simulink model "PHRControl"  (R2022a)
settings: Solver=FixedStepAuto  StartTime=0.0  StopTime=inf  FixedStep=.005  RelTol=1e-3
model workspace (MAT data in the model file):
  CPR = 10000
  amplitude = 0
  contactTime = 0
  desired_speed = 0
  equilibrium_length = 0
  h = 35
  hip_bend_factor = 0
  hip_fuzz = 0
  initHip = 0.523598775598
  initKnee = -1.0471975512
  k_landing_angle = 0
  k_slip = 0
  knee_bend_factor = 0
  knee_fuzz = 0
  lower_leg_length = 0.15
  max_torque = 8
  r = 1.35
  sample_time = [0 1]
  upper_leg_length = 0.15
  v_des = 0
  z_des = 0
undefined symbols (not defined in the file or in its folder): DiscIntNeverNeededParam, foot_x_flight, foot_y_flight, hasHopped, Hip_Impact_Angle, hip_range, Knee_Impact_Angle, Simscape_Transitions, simTime, SLIP_impact_angle
libraries: slpidlib x16, canmsglib x8, speedgoatlib_IO691 x7, simulink x2, slrealtimeutilitieslib x2
(part 3 of 3)

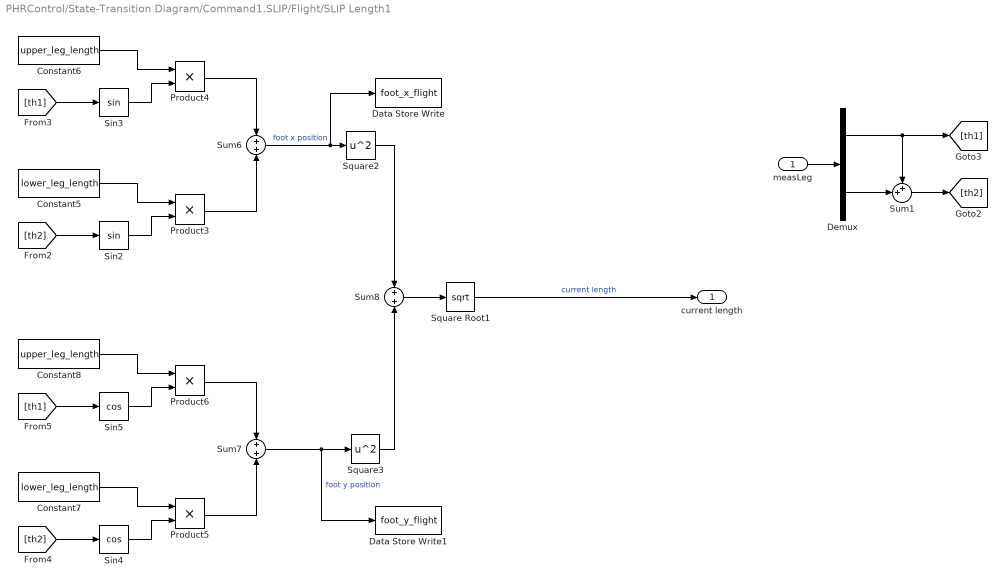
== system PHRControl/State-Transition Diagram/Command1.SLIP/Flight/SLIP Length1 ==
  measLeg : Inport
  Constant5 : Constant  Value=lower_leg_length
  Constant6 : Constant  Value=upper_leg_length
  Constant7 : Constant  Value=lower_leg_length
  Constant8 : Constant  Value=upper_leg_length
  Data Store Write : DataStoreWrite  DataStoreName=foot_x_flight  IndexOptions=Index vector (dialog)  Indices=1  OutputSizes=1
  Data Store Write1 : DataStoreWrite  DataStoreName=foot_y_flight  IndexOptions=Index vector (dialog)  Indices=1  OutputSizes=1
  Demux : Demux  Outputs=2
  Product{3..6} (4 alike) : Product
  Sin2 : Trigonometry
  Sin3 : Trigonometry
  Sin4 : Trigonometry  Operator=cos
  Sin5 : Trigonometry  Operator=cos
  Square Root1 : Sqrt
  Square2 : Math  Operator=square
  Square3 : Math  Operator=square
  Sum1 : Sum  Inputs=++|
  Sum6 : Sum  Inputs=+|+
  Sum7 : Sum  Inputs=+|+
  Sum8 : Sum  Inputs=+|+
  current length : Outport
  wires:
  Square2/1 -> Sum8/1
  Sum7/1 -> Data Store Write1/1, Square3/1  "foot y position"
  [th2] -> Sin2/1
  Square3/1 -> Sum8/2
  Sin4/1 -> Product5/2
  Constant5/1 -> Product3/1
  Constant7/1 -> Product5/1
  Product6/1 -> Sum7/1
  Product3/1 -> Sum6/2
  [th2] -> Sin4/1
  Product5/1 -> Sum7/2
  [th1] -> Sin5/1
  Sin3/1 -> Product4/2
  Constant8/1 -> Product6/1
  Sin5/1 -> Product6/2
  Sin2/1 -> Product3/2
  Sum6/1 -> Data Store Write/1, Square2/1  "foot x position"
  Constant6/1 -> Product4/1
  Product4/1 -> Sum6/1
  Sum8/1 -> Square Root1/1
  [th1] -> Sin3/1
  Square Root1/1 -> current length/1  "current length"
  Sum1/1 -> [th2]
  Demux/2 -> Sum1/2
  measLeg/1 -> Demux/1
  Demux/1 -> Sum1/1, [th1]

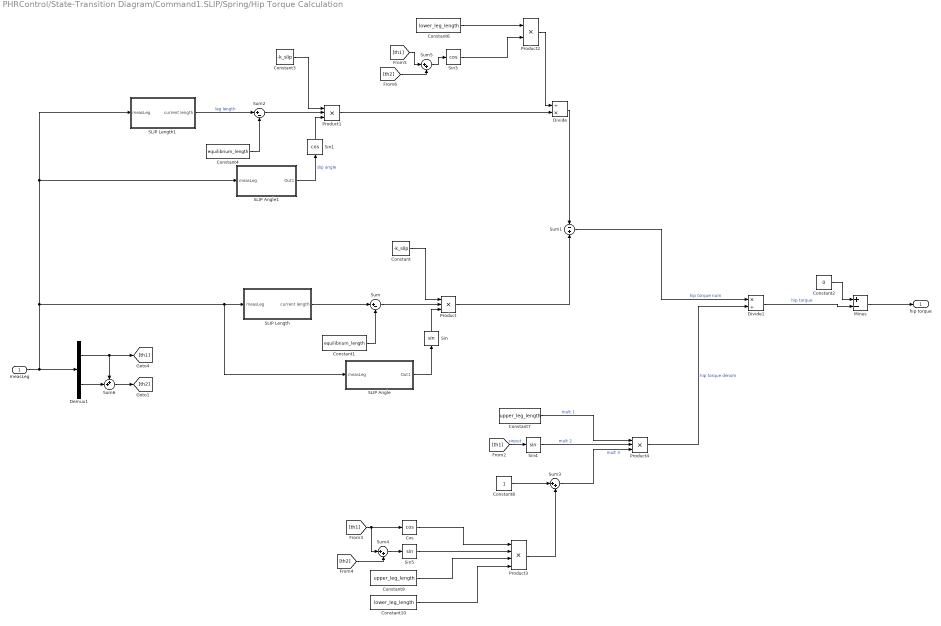
== system PHRControl/State-Transition Diagram/Command1.SLIP/Spring/Hip Torque Calculation ==
  measLeg : Inport
  Constant : Constant  Value=-k_slip
  Constant1 : Constant  Value=equilibrium_length
  Constant10 : Constant  Value=lower_leg_length
  Constant2 : Constant  Value=0
  Constant3 : Constant  Value=-k_slip
  Constant4 : Constant  Value=equilibrium_length
  Constant6 : Constant  Value=lower_leg_length
  Constant7 : Constant  Value=upper_leg_length
  Constant8 : Constant
  Constant9 : Constant  Value=upper_leg_length
  Cos : Trigonometry  Operator=cos
  Demux1 : Demux  Outputs=2
  Divide : Product  Inputs=/*
  Divide1 : Product  Inputs=*/
  Minus : Sum  Inputs=+-
  Product : Product  Inputs=3
  Product1 : Product  Inputs=3
  Product2 : Product
  Product3 : Product  Inputs=4
  Product4 : Product  Inputs=3
  SLIP Angle : Subsystem
  SLIP Angle1 : Subsystem
  SLIP Length : Subsystem
  SLIP Length1 : Subsystem
  Sin : Trigonometry
  Sin1 : Trigonometry  Operator=cos
  Sin3 : Trigonometry  Operator=cos
  Sin4 : Trigonometry
  Sin5 : Trigonometry
  Sum : Sum  Inputs=|+-
  Sum1 : Sum  Inputs=-|+
  Sum2 : Sum  Inputs=|+-
  Sum3 : Sum  Inputs=|++
  Sum4 : Sum  Inputs=|++
  Sum5 : Sum  Inputs=|++
  Sum6 : Sum  Inputs=++|
  hip torque : Outport
  wires:
  Sin1/1 -> Product1/3
  [th2] -> Sum4/2
  Constant/1 -> Product/1
  Sin5/1 -> Product3/2
  Constant7/1 -> Product4/1  "mult 1"
  Constant1/1 -> Sum/2
  Product2/1 -> Divide/1
  Product/1 -> Sum1/2
  Sin/1 -> Product/3
  Constant6/1 -> Product2/1
  Constant9/1 -> Product3/3
  Sum/1 -> Product/2
  Product3/1 -> Sum3/2
  Constant10/1 -> Product3/4
  SLIP Angle/1(Out1) -> Sin/1
  Sum1/1 -> Divide1/1  "hip torque num"
  Sum2/1 -> Product1/2
  Product4/1 -> Divide1/2  "hip torque denom"
  SLIP Length1/1(current length) -> Sum2/1  "leg length"
  Constant4/1 -> Sum2/2
  SLIP Angle1/1(Out1) -> Sin1/1  "slip angle"
  Divide1/1 -> Minus/2  "hip torque"
  Constant3/1 -> Product1/1
  Product1/1 -> Divide/2
  [th1] -> Sum4/1, Cos/1
  Sin3/1 -> Product2/2
  Sin4/1 -> Product4/2  "mult 2"
  Divide/1 -> Sum1/1
  SLIP Length/1(current length) -> Sum/1
  Sum3/1 -> Product4/3  "mult 3"
  [th1] -> Sin4/1  "sinput"
  Constant8/1 -> Sum3/1
  Cos/1 -> Product3/1
  Constant2/1 -> Minus/1
  Minus/1 -> hip torque/1
  Sum4/1 -> Sin5/1
  [th1] -> Sum5/1
  [th2] -> Sum5/2
  Sum5/1 -> Sin3/1
  Sum6/1 -> [th2]
  Demux1/2 -> Sum6/2
  measLeg/1 -> Demux1/1, SLIP Angle/1(measLeg), SLIP Length/1(measLeg), SLIP Angle1/1(measLeg), SLIP Length1/1(measLeg)
  Demux1/1 -> Sum6/1, [th1]

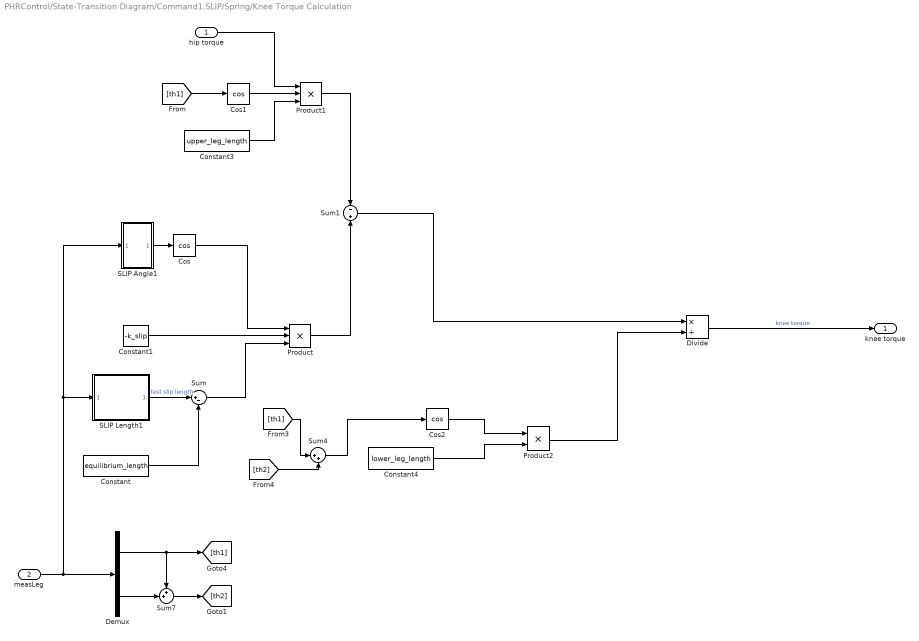
== system PHRControl/State-Transition Diagram/Command1.SLIP/Spring/Knee Torque Calculation ==
  hip torque : Inport
  measLeg : Inport  Port=2
  Constant : Constant  Value=equilibrium_length
  Constant1 : Constant  Value=-k_slip
  Constant3 : Constant  Value=upper_leg_length
  Constant4 : Constant  Value=lower_leg_length
  Cos : Trigonometry  Operator=cos
  Cos1 : Trigonometry  Operator=cos
  Cos2 : Trigonometry  Operator=cos
  Demux : Demux  Outputs=2
  Divide : Product  Inputs=*/
  Product : Product  Inputs=3
  Product1 : Product  Inputs=3
  Product2 : Product
  SLIP Angle1 : Subsystem
  SLIP Length1 : Subsystem
  Sum : Sum  Inputs=|+-
  Sum1 : Sum  Inputs=-|+
  Sum4 : Sum  Inputs=|++
  Sum7 : Sum  Inputs=++|
  knee torque : Outport
  wires:
  Constant3/1 -> Product1/3
  Constant/1 -> Sum/2
  Cos/1 -> Product/1
  Cos2/1 -> Product2/1
  SLIP Length1/1(current length) -> Sum/1  "test slip length"
  Sum1/1 -> Divide/1
  Constant4/1 -> Product2/2
  Product1/1 -> Sum1/1
  Constant1/1 -> Product/2
  [th1] -> Cos1/1
  Sum4/1 -> Cos2/1
  Cos1/1 -> Product1/2
  Product/1 -> Sum1/2
  SLIP Angle1/1(Out1) -> Cos/1
  Sum/1 -> Product/3
  Product2/1 -> Divide/2
  Divide/1 -> knee torque/1  "knee torque"
  hip torque/1 -> Product1/1
  [th1] -> Sum4/1
  [th2] -> Sum4/2
  Sum7/1 -> [th2]
  Demux/2 -> Sum7/2
  measLeg/1 -> Demux/1, SLIP Length1/1(measLeg), SLIP Angle1/1(measLeg)
  Demux/1 -> Sum7/1, [th1]

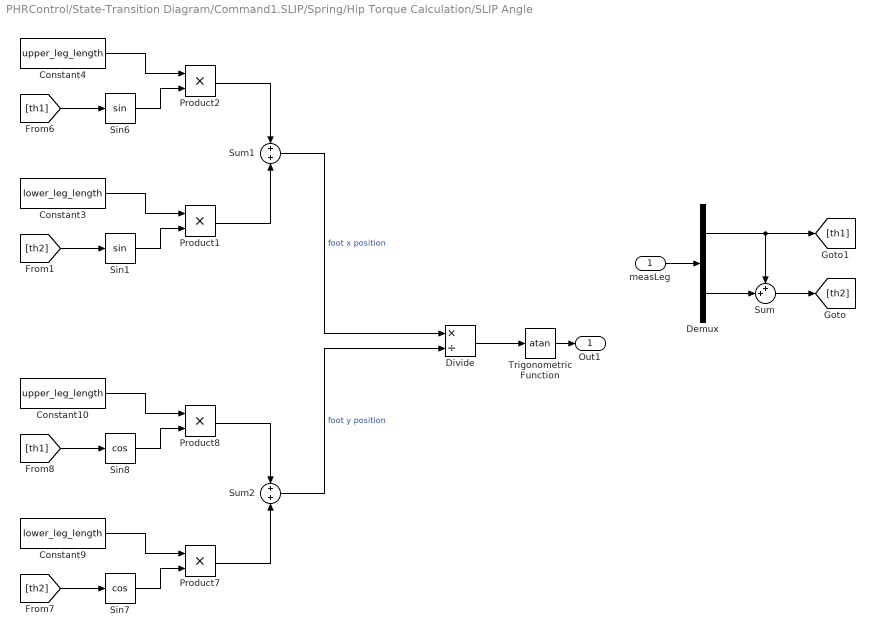
== system PHRControl/State-Transition Diagram/Command1.SLIP/Spring/Hip Torque Calculation/SLIP Angle ==
  measLeg : Inport
  Constant10 : Constant  Value=upper_leg_length
  Constant3 : Constant  Value=lower_leg_length
  Constant4 : Constant  Value=upper_leg_length
  Constant9 : Constant  Value=lower_leg_length
  Demux : Demux  Outputs=2
  Divide : Product  Inputs=*/
  Product{1..2,7..8} (4 alike) : Product
  Sin1 : Trigonometry
  Sin6 : Trigonometry
  Sin7 : Trigonometry  Operator=cos
  Sin8 : Trigonometry  Operator=cos
  Sum : Sum  Inputs=++|
  Sum1 : Sum  Inputs=+|+
  Sum2 : Sum  Inputs=+|+
  Trigonometric Function : Trigonometry  Operator=atan
  Out1 : Outport
  wires:
  Product2/1 -> Sum1/1
  Constant9/1 -> Product7/1
  Sin7/1 -> Product7/2
  Constant10/1 -> Product8/1
  Sin1/1 -> Product1/2
  [th1] -> Sin8/1
  Sin8/1 -> Product8/2
  Product7/1 -> Sum2/2
  [th2] -> Sin7/1
  Sum2/1 -> Divide/2  "foot y position"
  Trigonometric Function/1 -> Out1/1
  Product8/1 -> Sum2/1
  Sum1/1 -> Divide/1  "foot x position"
  Divide/1 -> Trigonometric Function/1
  [th1] -> Sin6/1
  Sin6/1 -> Product2/2
  [th2] -> Sin1/1
  Constant3/1 -> Product1/1
  Constant4/1 -> Product2/1
  Product1/1 -> Sum1/2
  Demux/1 -> Sum/1, [th1]
  Sum/1 -> [th2]
  measLeg/1 -> Demux/1
  Demux/2 -> Sum/2

== system PHRControl/State-Transition Diagram/Command1.SLIP/Spring/Hip Torque Calculation/SLIP Angle1 ==
  measLeg : Inport
  Constant10 : Constant  Value=upper_leg_length
  Constant3 : Constant  Value=lower_leg_length
  Constant4 : Constant  Value=upper_leg_length
  Constant9 : Constant  Value=lower_leg_length
  Demux : Demux  Outputs=2
  Divide : Product  Inputs=*/
  Product{1..2,7..8} (4 alike) : Product
  Sin1 : Trigonometry
  Sin6 : Trigonometry
  Sin7 : Trigonometry  Operator=cos
  Sin8 : Trigonometry  Operator=cos
  Sum : Sum  Inputs=++|
  Sum1 : Sum  Inputs=+|+
  Sum2 : Sum  Inputs=+|+
  Trigonometric Function : Trigonometry  Operator=atan
  Out1 : Outport
  wires:
  Product2/1 -> Sum1/1
  Constant9/1 -> Product7/1
  Sin7/1 -> Product7/2
  Constant10/1 -> Product8/1
  Sin1/1 -> Product1/2
  [th1] -> Sin8/1
  Sin8/1 -> Product8/2
  Product7/1 -> Sum2/2
  [th2] -> Sin7/1
  Sum2/1 -> Divide/2  "foot y position"
  Trigonometric Function/1 -> Out1/1
  Product8/1 -> Sum2/1
  Sum1/1 -> Divide/1  "foot x position"
  Divide/1 -> Trigonometric Function/1
  [th1] -> Sin6/1
  Sin6/1 -> Product2/2
  [th2] -> Sin1/1
  Constant3/1 -> Product1/1
  Constant4/1 -> Product2/1
  Product1/1 -> Sum1/2
  Demux/1 -> Sum/1, [th1]
  Demux/2 -> Sum/2
  Sum/1 -> [th2]
  measLeg/1 -> Demux/1

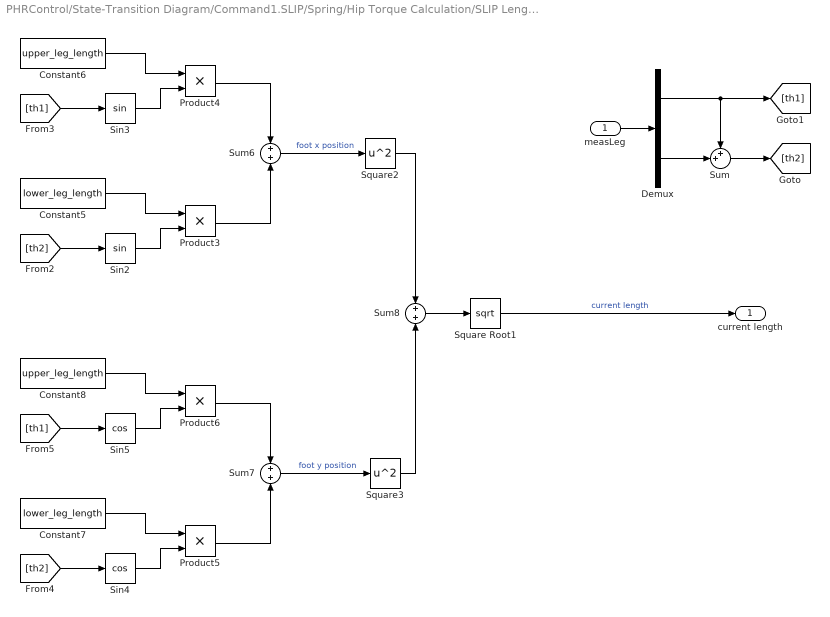
== system PHRControl/State-Transition Diagram/Command1.SLIP/Spring/Hip Torque Calculation/SLIP Length ==
  measLeg : Inport
  Constant5 : Constant  Value=lower_leg_length
  Constant6 : Constant  Value=upper_leg_length
  Constant7 : Constant  Value=lower_leg_length
  Constant8 : Constant  Value=upper_leg_length
  Demux : Demux  Outputs=2
  Product{3..6} (4 alike) : Product
  Sin2 : Trigonometry
  Sin3 : Trigonometry
  Sin4 : Trigonometry  Operator=cos
  Sin5 : Trigonometry  Operator=cos
  Square Root1 : Sqrt
  Square2 : Math  Operator=square
  Square3 : Math  Operator=square
  Sum : Sum  Inputs=++|
  Sum6 : Sum  Inputs=+|+
  Sum7 : Sum  Inputs=+|+
  Sum8 : Sum  Inputs=+|+
  current length : Outport
  wires:
  Square2/1 -> Sum8/1
  Sum7/1 -> Square3/1  "foot y position"
  [th2] -> Sin2/1
  Square3/1 -> Sum8/2
  Sin4/1 -> Product5/2
  Constant5/1 -> Product3/1
  Constant7/1 -> Product5/1
  Product6/1 -> Sum7/1
  Product3/1 -> Sum6/2
  [th2] -> Sin4/1
  Product5/1 -> Sum7/2
  [th1] -> Sin5/1
  Sin3/1 -> Product4/2
  Constant8/1 -> Product6/1
  Sin5/1 -> Product6/2
  Sin2/1 -> Product3/2
  Sum6/1 -> Square2/1  "foot x position"
  Constant6/1 -> Product4/1
  Product4/1 -> Sum6/1
  Sum8/1 -> Square Root1/1
  [th1] -> Sin3/1
  Square Root1/1 -> current length/1  "current length"
  Demux/1 -> Sum/1, [th1]
  Demux/2 -> Sum/2
  Sum/1 -> [th2]
  measLeg/1 -> Demux/1

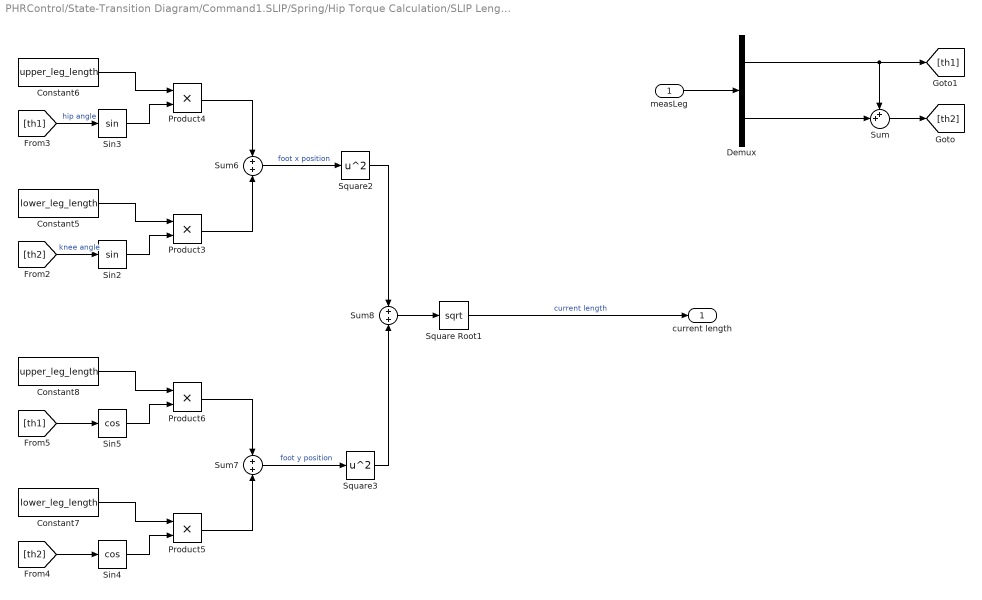
== system PHRControl/State-Transition Diagram/Command1.SLIP/Spring/Hip Torque Calculation/SLIP Length1 ==
  measLeg : Inport
  Constant5 : Constant  Value=lower_leg_length
  Constant6 : Constant  Value=upper_leg_length
  Constant7 : Constant  Value=lower_leg_length
  Constant8 : Constant  Value=upper_leg_length
  Demux : Demux  Outputs=2
  Product{3..6} (4 alike) : Product
  Sin2 : Trigonometry
  Sin3 : Trigonometry
  Sin4 : Trigonometry  Operator=cos
  Sin5 : Trigonometry  Operator=cos
  Square Root1 : Sqrt
  Square2 : Math  Operator=square
  Square3 : Math  Operator=square
  Sum : Sum  Inputs=++|
  Sum6 : Sum  Inputs=+|+
  Sum7 : Sum  Inputs=+|+
  Sum8 : Sum  Inputs=+|+
  current length : Outport
  wires:
  Square2/1 -> Sum8/1
  Sum7/1 -> Square3/1  "foot y position"
  [th2] -> Sin2/1  "knee angle"
  Square3/1 -> Sum8/2
  Sin4/1 -> Product5/2
  Constant5/1 -> Product3/1
  Constant7/1 -> Product5/1
  Product6/1 -> Sum7/1
  Product3/1 -> Sum6/2
  [th2] -> Sin4/1
  Product5/1 -> Sum7/2
  [th1] -> Sin5/1
  Sin3/1 -> Product4/2
  Constant8/1 -> Product6/1
  Sin5/1 -> Product6/2
  Sin2/1 -> Product3/2
  Sum6/1 -> Square2/1  "foot x position"
  Constant6/1 -> Product4/1
  Product4/1 -> Sum6/1
  Sum8/1 -> Square Root1/1
  [th1] -> Sin3/1  "hip angle"
  Square Root1/1 -> current length/1  "current length"
  measLeg/1 -> Demux/1
  Sum/1 -> [th2]
  Demux/1 -> Sum/1, [th1]
  Demux/2 -> Sum/2

== system PHRControl/State-Transition Diagram/Command1.SLIP/Spring/Knee Torque Calculation/SLIP Angle1 ==
  measLeg : Inport
  Constant10 : Constant  Value=upper_leg_length
  Constant3 : Constant  Value=lower_leg_length
  Constant4 : Constant  Value=upper_leg_length
  Constant9 : Constant  Value=lower_leg_length
  Demux : Demux  Outputs=2
  Divide : Product  Inputs=*/
  Product{1..2,7..8} (4 alike) : Product
  Sin1 : Trigonometry
  Sin6 : Trigonometry
  Sin7 : Trigonometry  Operator=cos
  Sin8 : Trigonometry  Operator=cos
  Sum1 : Sum  Inputs=+|+
  Sum2 : Sum  Inputs=+|+
  Sum7 : Sum  Inputs=++|
  Trigonometric Function : Trigonometry  Operator=atan
  Out1 : Outport
  wires:
  Product2/1 -> Sum1/1
  Constant9/1 -> Product7/1
  Sin7/1 -> Product7/2
  Constant10/1 -> Product8/1
  Sin1/1 -> Product1/2
  [th1] -> Sin8/1
  Sin8/1 -> Product8/2
  Product7/1 -> Sum2/2
  [th2] -> Sin7/1
  Sum2/1 -> Divide/2  "foot y position"
  Trigonometric Function/1 -> Out1/1
  Product8/1 -> Sum2/1
  Sum1/1 -> Divide/1  "foot x position"
  Divide/1 -> Trigonometric Function/1
  [th1] -> Sin6/1
  Sin6/1 -> Product2/2
  [th2] -> Sin1/1
  Constant3/1 -> Product1/1
  Constant4/1 -> Product2/1
  Product1/1 -> Sum1/2
  Sum7/1 -> [th2]
  Demux/2 -> Sum7/2
  measLeg/1 -> Demux/1
  Demux/1 -> Sum7/1, [th1]

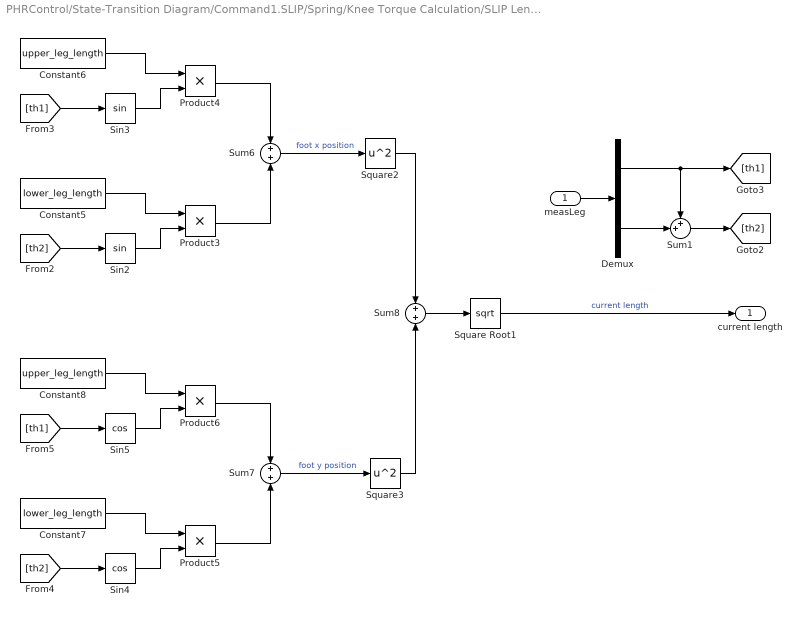
== system PHRControl/State-Transition Diagram/Command1.SLIP/Spring/Knee Torque Calculation/SLIP Length1 ==
  measLeg : Inport
  Constant5 : Constant  Value=lower_leg_length
  Constant6 : Constant  Value=upper_leg_length
  Constant7 : Constant  Value=lower_leg_length
  Constant8 : Constant  Value=upper_leg_length
  Demux : Demux  Outputs=2
  Product{3..6} (4 alike) : Product
  Sin2 : Trigonometry
  Sin3 : Trigonometry
  Sin4 : Trigonometry  Operator=cos
  Sin5 : Trigonometry  Operator=cos
  Square Root1 : Sqrt
  Square2 : Math  Operator=square
  Square3 : Math  Operator=square
  Sum1 : Sum  Inputs=++|
  Sum6 : Sum  Inputs=+|+
  Sum7 : Sum  Inputs=+|+
  Sum8 : Sum  Inputs=+|+
  current length : Outport
  wires:
  Square2/1 -> Sum8/1
  Sum7/1 -> Square3/1  "foot y position"
  [th2] -> Sin2/1
  Square3/1 -> Sum8/2
  Sin4/1 -> Product5/2
  Constant5/1 -> Product3/1
  Constant7/1 -> Product5/1
  Product6/1 -> Sum7/1
  Product3/1 -> Sum6/2
  [th2] -> Sin4/1
  Product5/1 -> Sum7/2
  [th1] -> Sin5/1
  Sin3/1 -> Product4/2
  Constant8/1 -> Product6/1
  Sin5/1 -> Product6/2
  Sin2/1 -> Product3/2
  Sum6/1 -> Square2/1  "foot x position"
  Constant6/1 -> Product4/1
  Product4/1 -> Sum6/1
  Sum8/1 -> Square Root1/1
  [th1] -> Sin3/1
  Square Root1/1 -> current length/1  "current length"
  Sum1/1 -> [th2]
  Demux/2 -> Sum1/2
  measLeg/1 -> Demux/1
  Demux/1 -> Sum1/1, [th1]

== matlab function PHRControl/Read All/If Action Subsystem2/Encoder 1 to Vertical Data ==
  data: th1Raw input; z output; thd1Raw input; zd output; CPR parameter; r parameter; h parameter
function [z, zd] = Enc1ToVert(th1Raw, thd1Raw, CPR, r, h)

th1 = th1Raw*2*pi/(4*CPR);
thd1 = thd1Raw*2*pi/(4*CPR);
    
z = r*sin(th1)+h;
zd = thd1*r*cos(th1);

end

== stateflow chart PHRControl/State-Transition Diagram/Command1.SLIP ==
  state Flight
  state Unload
  state Load
  state Idle
  state Spring
  Unload -> Flight : [after(5,msec)]{contactTime = simTime(end)-landingTime,n=n+1,hasHopped = 1}
  Flight -> Load : [Simscape_Transitions == true]{SLIP_impact_angle = atan(foot_x_flight(end)/foot_y_flight(end)),landingTime=simTime(end)}
  (default) -> Idle : {n=0, contactTime = 0,hasHopped = 0,landingTime = 0}
  Load -> Idle [order 2] : [run == 0]
  Idle -> Load : [run == 1]
  Spring -> Unload : [Simscape_Transitions == false]
  Load -> Spring [order 1] : [after(5,msec)]
  data: sf_internal_action_state_placeholder_data local double size=1 =0; sf_internal_action_state_placeholder_data local double size=1 =0; sf_internal_action_state_placeholder_data local double size=1 =0; sf_internal_action_state_placeholder_data local double size=1 =0; sf_internal_action_state_placeholder_data local double size=1 =0; measLeg input; contactTime data_store_memory; Simscape_Transitions data_store_memory; Machine_State output double size=1; n output double size=1; foot_x_flight data_store_memory; foot_y_flight data_store_memory; SLIP_impact_angle data_store_memory; simTime data_store_memory; landingTime local; hasHopped data_store_memory; run data_store_memory; T1 output double size=1; T2 output double size=1; Xd input

== stateflow chart PHRControl/State-Transition Diagram/Command1.Raibert ==
  state Flight
  state Unload
  state Load
  state Idle
  state Thrust
  state Compress
  Unload -> Flight : [after(5,msec)]{contactTime = simTime - landingTime,hasHopped = 1}
  Flight -> Load : [Simscape_Transitions == true]{landingTime = simTime,Hip_Impact_Angle = measLeg(1,end),Knee_Impact_Angle = measLeg(2,end)}
  (default) -> Idle : {contactTime = 0,hasHopped = 0,landingTime = 0}
  Load -> Idle [order 2] : [run == 0]
  Idle -> Load : [run == 1]
  Thrust -> Unload : [Simscape_Transitions == false]
  Load -> Compress [order 1] : [after(5,msec)]
  Compress -> Thrust : [((1+hip_range)*abs(abs(Hip_Impact_Angle)-hip_bend_factor)>abs(measLeg(1)))&&(abs(measLeg(1))>(1-hip_range)*abs(abs(Hip_Impact_Angle)-hip_bend_factor))]
  data: sf_internal_action_state_placeholder_data local double size=1 =0; sf_internal_action_state_placeholder_data local double size=1 =0; sf_internal_action_state_placeholder_data local double size=1 =0; sf_internal_action_state_placeholder_data local double size=1 =0; sf_internal_action_state_placeholder_data local double size=1 =0; sf_internal_action_state_placeholder_data local double size=1 =0; measLeg input; contactTime local double; Machine_State output double size=1; Knee_Impact_Angle data_store_memory; Hip_Impact_Angle data_store_memory; hip_range data_store_memory; hasHopped data_store_memory; hip_bend_factor data_store_memory; landingTime local; simTime data_store_memory; run data_store_memory; T2 output double size=1; T1 output double size=1; Xd input; Simscape_Transitions data_store_memory

== stateflow chart PHRControl/State-Transition Diagram/Command1.HSW_Controller ==
  state Flight
  state Unload
  state Load
  state Idle
  state HSW
  Unload -> Flight : [after(5,msec)]{contactTime = simTime(end)-landingTime,hasHopped=1}
  Flight -> Load : [Simscape_Transitions == true]{SLIP_impact_angle = atan(foot_x_flight(end)/foot_y_flight(end)),landingTime = simTime(end)}
  (default) -> Idle : {contactTime = 0,hasHopped = 0,landingTime = 0}
  Load -> Idle [order 2] : [run == 0]
  Idle -> Load : [run == 1]
  HSW -> Unload : [Simscape_Transitions == false]
  Load -> HSW [order 1] : [after(5,msec)]
  data: sf_internal_action_state_placeholder_data local double size=1 =0; sf_internal_action_state_placeholder_data local double size=1 =0; sf_internal_action_state_placeholder_data local double size=1 =0; sf_internal_action_state_placeholder_data local double size=1 =0; sf_internal_action_state_placeholder_data local double size=1 =0; measLeg input; contactTime data_store_memory; Simscape_Transitions data_store_memory; Machine_State output double size=1; SLIP_impact_angle data_store_memory; foot_x_flight data_store_memory; foot_y_flight data_store_memory; simTime data_store_memory; landingTime local; hasHopped data_store_memory; run data_store_memory; T1 output double size=1; Xd input; T2 output double size=1; Z input

== matlab function PHRControl/Danger Detector Function ==
  data: P1 input; danger output; P2 input
function danger = isDanger(P1, P2)
    % Pmux position matrix radians
    %       [p(ID1),p(ID2),p(ID3),p(IDN)]

    
    p1Max = 6; 
    %p1Min = -2;
    p2Max = 2;
    %p2Min = -2;
       
    danger = 0;
    %if((0<sum([P1>p1Max] + [P1<p1Min] - [P1<=-95.5])) || (0<sum([P2>p2Max] + [P2<p2Min] - [P2<=-95.5])))
    if abs(P2) > p2Max || abs(P1) > p1Max
    
%     if((0<sum([P1>p1Max] + [P1<p1Min])) || (0<sum([P2>p2Max] + [P2<p2Min])))
        danger = 1;
    end

== matlab function PHRControl/State-Transition Diagram/Command1.HSW_Controller/HSW/Sine Generator ==
  data: t input; HSW output; contactTime input; amplitude input
function HSW= fcn(t,contactTime,amplitude)

if contactTime ~= 0
HSW = amplitude*sin(pi*t/contactTime);
else
HSW = .3*sin(pi*t/.3);
end

end

== stateflow chart PHRControl/State-Transition Diagram ==
  state Start
  note: Simulink State Transition Diagram
      | "IsReady" is a user defined varable that controls the flow through the Finite State Mechine
      | Commands: 0. Zero
      | 1. Init
      | 2. Stand
      | 3. Raibert
      | 5. HSW
      | 6. SLIP
      | 7. Jump
      | 4. Deinit
  state Zero
    entry:
    c = 1;
  state Init
    entry:
    c = 2;
  state SlowDown
    entry:
    %deinitiate mode
    c = 4
  state Command1
    entry:
    c = 3;
    state Raibert
    state Stand
      entry:
      during:
      theta1 = initHip;
      theta2 = initKnee;
      Kp1 = 30;
      Kp2 = 30;
      Kd1 = 0.2;
      Kd2 = 0.2;
      T1 = 0;
      T2 = 0;
    state SLIP
    state Flight
      entry:
      during:
      theta1 = initHip;
      theta2 = initKnee;
      Kp1 = 4;
      Kp2 = 4;
      Kd1 = 0.5;
      Kd2 = 0.5;
    state Stance
      entry:
      during:
      T1 = 5
      T2 = 5
    state HSW_Controller
    Command1.Stand -> Raibert [order 2] : [isReady == 3]
        | {Kp1 = 0, Kp2 = 0, Kd1 = 0, Kd2 = 0}
    Raibert -> Command1.Stand : [MachineState == 0 & isReady == 2]
    (default) -> Command1.Stand
    Command1.Stand -> SLIP [order 1] : [isReady == 6]
        | {Kp1 = 0, Kp2 = 0, Kd1 = 0, Kd2 = 0}
    Flight -> Stance : [Simscape_Transitions == true]
        | {Kp1 = 0, Kp2 = 0, Kd1 = 0, Kd2 = 0}
    Stance -> Command1.Stand [order 2] : [isReady == 2]
    Command1.Stand -> Stance [order 4] : [isReady == 7]
        | {Kp1 = 0, Kp2 = 0, Kd1 = 0, Kd2 = 0}
    SLIP -> Command1.Stand : [MachineState == 0 & isReady == 2]
    Stance -> Flight [order 1] : [Simscape_Transitions == false]
        | {T1 = 0, T2 = 0}
    Command1.Stand -> HSW_Controller [order 3] : [isReady == 5]
        | {Kp1 = 0, Kp2 = 0, Kd1 = 0, Kd2 =0}
    HSW_Controller -> Command1.Stand : [MachineState == 0 & isReady == 2]
  state FinalShutdown
    entry:
    Kp1 = 0;
    Kp2 = 0;
    theta1 = 0;
    theta2 = 0;
    T1 = 0;
    T2 = 0;
    Kd1 = .1;
    Kd2 = .1;
  state Deinitiate
    entry:
    c = 4;
  state Command [commented out]
    entry:
    c = 3;
    p_sit = -.8;
    p_stand = -1.35;
    p_jump = -.4;
    state JumpPrep [commented out]
      entry:
      to = t;
      % Left Side
      theta1 = pc;
      po1 = theta1;
      slope1 = (pf - po1)/tstep;
      theta2 = pc2;
      po2 = theta2;
      slope2 = (Th2Th1*pf - po2)/tstep;
      %Right Side
      theta1r = pcr;
      po1r = theta1r;
      slope1r = (pfr - po1r)/tstep;
      theta2r = pc2r;
      po2r = theta2r;
      slope2r = (Th2Th1*pfr - po2r)/tstep;
      during:
      theta1  = po1  + slope1*(t-to);
      theta2  = po2  + slope2*(t-to);
      theta1r = po1r + slope1r*(t-to);
      theta2r = po2r + slope2r*(t-to);
    state Stand [commented out]
      entry:
      to = t;
      % Left Side
      theta1 = pc;
      po1 = theta1;
      slope1 = (pf - po1)/tstep;
      theta2 = pc2;
      po2 = theta2;
      slope2 = (Th2Th1*pf - po2)/tstep;
      %Right Side
      theta1r = pcr;
      po1r = theta1r;
      slope1r = (pfr - po1r)/tstep;
      theta2r = pc2r;
      po2r = theta2r;
      slope2r = (Th2Th1*pfr - po2r)/tstep;
      during:
      theta1  = po1  + slope1*(t-to);
      theta2  = po2  + slope2*(t-to);
      theta1r = po1r + slope1r*(t-to);
      theta2r = po2r + slope2r*(t-to);
    state Jump [commented out]
      entry:
      to = t;
      % Left Side
      theta1 = pc;
      po1 = theta1;
      slope1 = (pf - po1)/tjump;
      theta2 = pc2;
      po2 = theta2;
      slope2 = (Th2Th1*pf - po2)/tjump;
      %Right Side
      theta1r = pcr;
      po1r = theta1r;
      slope1r = (pfr - po1r)/tjump;
      theta2r = pc2r;
      po2r = theta2r;
      slope2r = (Th2Th1*pfr - po2r)/tjump;
      during:
      theta1  = po1  + slope1*(t-to);
      theta2  = po2  + slope2*(t-to);
      theta1r = po1r + slope1r*(t-to);
      theta2r = po2r + slope2r*(t-to);
    state Idle [commented out]
    state Land [commented out]
      entry:
      to = t;
      Kp1temp = Kp1
      Kp2temp = Kp2
      Kp1 = 15;
      Kp2 = 15;
      % Left Side
      theta1 = pc;
      po1 = theta1;
      slope1 = (pf - po1)/tjump;
      theta2 = pc2;
      po2 = theta2;
      slope2 = (Th2Th1*pf - po2)/tjump;
      %Right Side
      theta1r = pcr;
      po1r = theta1r;
      slope1r = (pfr - po1r)/tjump;
      theta2r = pc2r;
      po2r = theta2r;
      slope2r = (Th2Th1*pfr - po2r)/tjump;
      during:
      theta1  = po1  + slope1*(t-to);
      theta2  = po2  + slope2*(t-to);
      theta1r = po1r + slope1r*(t-to);
      theta2r = po2r + slope2r*(t-to);
    state LeftUp [commented out]
      entry:
      to = t;
      % Left Side
      theta1 = pc;
      po1 = theta1;
      slope1 = (pf - po1)/tstep;
      theta2 = pc2;
      po2 = theta2;
      slope2 = (Th2Th1*pf - po2)/tstep;
      %Right Side
      theta1r = pcr;
      po1r = theta1r;
      slope1r = (pfr - po1r)/tstep;
      theta2r = pc2r;
      po2r = theta2r;
      slope2r = (Th2Th1*pfr - po2r)/tstep;
      during:
      theta1  = po1  + slope1*(t-to);
      theta2  = po2  + slope2*(t-to);
      theta1r = po1r + slope1r*(t-to);
      theta2r = po2r + slope2r*(t-to);
    state RightUp [commented out]
      entry:
      to = t;
      % Left Side
      theta1 = pc;
      po1 = theta1;
      slope1 = (pf - po1)/tstep;
      theta2 = pc2;
      po2 = theta2;
      slope2 = (Th2Th1*pf - po2)/tstep;
      %Right Side
      theta1r = pcr;
      po1r = theta1r;
      slope1r = (pfr - po1r)/tstep;
      theta2r = pc2r;
      po2r = theta2r;
      slope2r = (Th2Th1*pfr - po2r)/tstep;
      during:
      theta1  = po1  + slope1*(t-to);
      theta2  = po2  + slope2*(t-to);
      theta1r = po1r + slope1r*(t-to);
      theta2r = po2r + slope2r*(t-to);
    state Sit [commented out]
      entry:
      to = t;
      % Left Side
      theta1 = pc;
      po1 = theta1;
      slope1 = (pf - po1)/tstep;
      theta2 = pc2;
      po2 = theta2;
      slope2 = (Th2Th1*pf - po2)/tstep;
      %Right Side
      theta1r = pcr;
      po1r = theta1r;
      slope1r = (pfr - po1r)/tstep;
      theta2r = pc2r;
      po2r = theta2r;
      slope2r = (Th2Th1*pfr - po2r)/tstep;
      during:
      theta1  = po1  + slope1*(t-to);
      theta2  = po2  + slope2*(t-to);
      theta1r = po1r + slope1r*(t-to);
      theta2r = po2r + slope2r*(t-to);
    state Idle1 [commented out]
      exit:
      Kp1 = Kp1temp;
      Kp2 = Kp2temp;
    (default) -> Command.Stand [commented out] : {pf = p_sit; pfr = p_sit;}
    Command.Stand -> Idle [commented out] : [(theta1 >= pf & slope1>0) | (theta1 <= pf & slope1<0) & (theta1r >= pfr & slope1r>0) | (theta1r <= pfr & slope1r<0)]
        | {theta1 = pf; theta2 = theta1 * Th2Th1; theta1r = pfr; theta2r = theta1r * Th2Th1;}
    Idle -> Command.Stand [commented out] : [wasReady ~= isReady & isReady == 2]
        | {pf = p_sit; pfr = p_sit; wasReady = isReady;}
    Idle -> JumpPrep [commented out] : [wasReady ~= isReady & isReady == 8]
        | {pf = p_mid; pfr = p_mid; wasReady = isReady;}
    JumpPrep -> Idle [commented out] : [(theta1 >= pf & slope1>0) | (theta1 <= pf & slope1<0) & (theta1r >= pfr & slope1r>0) | (theta1r <= pfr & slope1r<0)]
        | {theta1 = pf; theta2 = theta1 * Th2Th1; theta1r = pfr; theta2r = theta1r * Th2Th1;}
    Idle -> Jump [commented out] : [wasReady == 8 & isReady == 7]{pf = p_jump; pfr = p_jump; wasReady = isReady;}
    Idle1 -> Idle [commented out] : [wasReady ~= isReady]
    Idle -> LeftUp [commented out] : [wasReady ~= isReady & isReady == 6]
        | {pf = p_sit; pfr = p_mid; wasReady = isReady;}
    LeftUp -> Idle [commented out] : [(theta1 >= pf & slope1>0) | (theta1 <= pf & slope1<0) & (theta1r >= pfr & slope1r>0) | (theta1r <= pfr & slope1r<0)]
        | {theta1 = pf; theta2 = theta1 * Th2Th1; theta1r = pfr; theta2r = theta1r * Th2Th1;}
    RightUp -> Idle [commented out] : [(theta1 >= pf & slope1>0) | (theta1 <= pf & slope1<0) & (theta1r >= pfr & slope1r>0) | (theta1r <= pfr & slope1r<0)]
        | {theta1 = pf; theta2 = theta1 * Th2Th1; theta1r = pfr; theta2r = theta1r * Th2Th1;}
    Idle -> RightUp [commented out] : [wasReady ~= isReady & isReady == 5]
        | {pf = p_mid; pfr = p_sit; wasReady = isReady;}
    Sit -> Idle [commented out] : [(theta1 >= pf & slope1>0) | (theta1 <= pf & slope1<0) & (theta1r >= pfr & slope1r>0) | (theta1r <= pfr & slope1r<0)]
        | {theta1 = pf; theta2 = theta1 * Th2Th1; theta1r = pfr; theta2r = theta1r * Th2Th1;}
    Idle -> Sit [commented out] : [wasReady ~= isReady & isReady == 3]
        | {pf = p_stand; pfr = p_stand; wasReady = isReady;}
    Jump -> Land [commented out] : [(theta1 >= pf & slope1>0) | (theta1 <= pf & slope1<0) & (theta1r >= pfr & slope1r>0) | (theta1r <= pfr & slope1r<0)]
        | {theta1 = pf; theta2 = theta1 * Th2Th1; theta1r = pfr; theta2r = theta1r * Th2Th1; pf = p_sit; pfr = p_sit;}
    Land -> Idle1 [commented out] : [(theta1 >= pf & slope1>0) | (theta1 <= pf & slope1<0) & (theta1r >= pfr & slope1r>0) | (theta1r <= pfr & slope1r<0)]
        | {theta1 = pf; theta2 = theta1 * Th2Th1; theta1r = pfr; theta2r = theta1r * Th2Th1;}
  (default) -> Start
  Start -> Init [order 2] : [isReady == 1]
  Start -> Zero [order 1] : [isReady == 0]
  SlowDown -> Zero [order 2] : [after(1,sec) & ~(theta1 == theta2) ]
  Zero -> SlowDown
  SlowDown -> Init [order 1] : [isReady == 1]
  Init -> FinalShutdown [order 1] : [isReady == 4 | danger == 1]
  Init -> Command1 [order 2] : [isReady == 2]
  Command1 -> FinalShutdown : [isReady == 4 | danger == 1]
  FinalShutdown -> Deinitiate
  Deinitiate -> (junction 36) : after(3,sec)
  (junction 36) -> Deinitiate : {stop = 1;}
  data: n output double size=1; MachineState output double size=1; stop output =0; theta1 output; theta2 output; c output; T1 output double size=1; T2 output double size=1; Kp1 output =5; Kp2 output =5; Kd1 output =.4; Kd2 output =.4; danger input; isReady input; Xd input; Z input; measLeg input; Simscape_Transitions data_store_memory; Hip_Impact_Angle data_store_memory; Knee_Impact_Angle data_store_memory; hasHopped data_store_memory; hip_bend_factor data_store_memory; hip_range data_store_memory; run data_store_memory; simTime data_store_memory; SLIP_impact_angle data_store_memory; contactTime data_store_memory; foot_x_flight data_store_memory; foot_y_flight data_store_memory; initHip parameter; initKnee parameter

== matlab function PHRControl/State-Transition Diagram/Command1.HSW_Controller/HSW/Torque Calculator ==
  data: FGy input; FGx input; th1 input; th2 input; T1 output; upper_leg_length parameter; T2 output; lower_leg_length parameter
function [T1, T2] = fcn(FGy, FGx, th1, th2, upper_leg_length, lower_leg_length)

% Define shorthand for sines and cosines
s1 = sin(th1);
c1 = cos(th1);
s12 = sin(th1+th2);
c12 = cos(th1+th2);

% Define Jacobian
J = [-upper_leg_length*s1-lower_leg_length*s12    -lower_leg_length*s12
      upper_leg_length*c1+lower_leg_length*c12     lower_leg_length*c12];

% Find Torques
T = J'*[FGx; FGy];

T(1) = -T(1);

T1 = T(1);
T2 = T(2);
%T_transp = transpose(T);

end

== matlab function PHRControl/Collision Detector ==
  data: pastground input; dI1 input; ground output; dI2 input
function ground = fcn(pastground, dI1, dI2)

dI1 = abs(dI1);
dI2 = abs(dI2);

maxCur = max(dI1, dI2);

if maxCur > 50
    if pastground == true
        ground = false;
    else
        ground = true;
    end
else
    ground = pastground;
end

== matlab function PHRControl/Read All/If Action Subsystem1/Encoder 2 to Vertical Data ==
  data: th2Raw input; x output; thd2Raw input; xd output; r parameter; CPR parameter
function [x, xd] = Enc2ToVert(th2Raw, thd2Raw, r, CPR)

th2= th2Raw*2*pi/(4*CPR);
thd2 = thd2Raw/1000;

x = r*sin(th2);
xd = thd2*r*cos(th2);

end

== matlab function PHRControl/Read All/If Action Subsystem3/bytes -> floats ==
  data: position input; position output; velocity output; I_ff output; velocity input; I_ff input
function [position, velocity, I_ff] = fcn(position, velocity, I_ff)

P_MIN  =-95.5;  % [rad]
P_MAX  = 95.5;  % [rad]
V_MIN  =-45;    % [rad/s]
V_MAX  = 45;    % [rad/s]
I_MIN  =-40;    % []
I_MAX  = 40;    % []

position = position*(P_MAX  - P_MIN)/65535+ P_MIN;
velocity = velocity*(V_MAX  - V_MIN)/4095 + V_MIN;
I_ff     = I_ff*(I_MAX  - I_MIN)/4095 + I_MIN;

== matlab function PHRControl/ID2 Write Knee Data/floats -> bytes ==
  data: position input; b output uint8 size=8; velocity input; K_p input; K_d input; T_ff input
function b = fcn(position, velocity, K_p, K_d, T_ff)

P_MIN  =-95.5;  % [rad]
P_MAX  = 95.5;  % [rad]
V_MIN  =-45;    % [rad/s] 30 to 45
V_MAX  = 45;    % [rad/s]
KP_MIN = 0;     % [Nm/rad]
KP_MAX = 500;   % [Nm/rad]
KD_MIN = 0;     % [Nm*s/rad
KD_MAX = 5;     % [Nm*s/rad
T_MIN  =-18;    % [Nm]
T_MAX  = 18;    % [Nm]

position = floor((max(min(position,P_MAX) ,P_MIN)  - P_MIN )*65535/(P_MAX  - P_MIN));
velocity = floor((max(min(velocity,V_MAX) ,V_MIN)  - V_MIN )*4095 /(V_MAX  - V_MIN));
K_p      = floor((max(min(K_p     ,KP_MAX),KP_MIN) - KP_MIN)*4095 /(KP_MAX - KP_MIN));
K_d      = floor((max(min(K_d     ,V_MAX) ,V_MIN)  - KD_MIN)*4095 /(KD_MAX - KD_MIN));
T_ff     = floor((max(min(T_ff    ,V_MAX) ,V_MIN)  - T_MIN )*4095 /(T_MAX  - T_MIN));

p  = dec2bin(position);
p  = [repmat('0', 1, 16-length(p)),p];
v  = dec2bin(velocity);
v  = [repmat('0', 1, 12-length(v)),v];
kp = dec2bin(K_p);
kp  = [repmat('0', 1, 12-length(kp)),kp];
kd = dec2bin(K_d);
kd  = [repmat('0', 1, 12-length(kd)),kd];
t  = dec2bin(T_ff);
t  = [repmat('0', 1, 12-length(t)),t];

B = repmat('0', 8, 8);

B(1,:) = p(1:8);
B(2,:) = p(9:16);
B(3,:) = v(1:8);
B(4,:) = [v(9:12),kp(1:4)];
B(5,:) = kp(5:12);
B(6,:) = kd(1:8);
B(7,:) = [kd(9:12),t(1:4)];
B(8,:) = t(5:12);

B  = bin2dec(B);

b = uint8(B);

== matlab function PHRControl/ID1 Write Hip Data/floats -> bytes ==
  data: position input; b output uint8 size=8; velocity input; K_p input; K_d input; T_ff input
function b = fcn(position, velocity, K_p, K_d, T_ff)

P_MIN  =-95.5;  % [rad]
P_MAX  = 95.5;  % [rad]
V_MIN  =-45;    % [rad/s] 30 to 45
V_MAX  = 45;    % [rad/s]
KP_MIN = 0;     % [Nm/rad]
KP_MAX = 500;   % [Nm/rad]
KD_MIN = 0;     % [Nm*s/rad
KD_MAX = 5;     % [Nm*s/rad
T_MIN  =-18;    % [Nm]
T_MAX  = 18;    % [Nm]

position = floor((max(min(position,P_MAX) ,P_MIN)  - P_MIN )*65535/(P_MAX  - P_MIN));
velocity = floor((max(min(velocity,V_MAX) ,V_MIN)  - V_MIN )*4095 /(V_MAX  - V_MIN));
K_p      = floor((max(min(K_p     ,KP_MAX),KP_MIN) - KP_MIN)*4095 /(KP_MAX - KP_MIN));
K_d      = floor((max(min(K_d     ,V_MAX) ,V_MIN)  - KD_MIN)*4095 /(KD_MAX - KD_MIN));
T_ff     = floor((max(min(T_ff    ,V_MAX) ,V_MIN)  - T_MIN )*4095 /(T_MAX  - T_MIN));

p  = dec2bin(position);
p  = [repmat('0', 1, 16-length(p)),p];
v  = dec2bin(velocity);
v  = [repmat('0', 1, 12-length(v)),v];
kp = dec2bin(K_p);
kp  = [repmat('0', 1, 12-length(kp)),kp];
kd = dec2bin(K_d);
kd  = [repmat('0', 1, 12-length(kd)),kd];
t  = dec2bin(T_ff);
t  = [repmat('0', 1, 12-length(t)),t];

B = repmat('0', 8, 8);

B(1,:) = p(1:8);
B(2,:) = p(9:16);
B(3,:) = v(1:8);
B(4,:) = [v(9:12),kp(1:4)];
B(5,:) = kp(5:12);
B(6,:) = kd(1:8);
B(7,:) = [kd(9:12),t(1:4)];
B(8,:) = t(5:12);

B  = bin2dec(B);

b = uint8(B);

== matlab function PHRControl/Read All/If Action Subsystem4/bytes -> floats ==
  data: position input; position output; velocity output; I_ff output; velocity input; I_ff input
function [position, velocity, I_ff] = fcn(position, velocity, I_ff)

P_MIN  =-95.5;  % [rad]
P_MAX  = 95.5;  % [rad]
V_MIN  =-45;    % [rad/s]
V_MAX  = 45;    % [rad/s]
I_MIN  =-40;    % []
I_MAX  = 40;    % []

position = position*(P_MAX  - P_MIN)/65535+ P_MIN;
velocity = velocity*(V_MAX  - V_MIN)/4095 + V_MIN;
I_ff     = I_ff*(I_MAX  - I_MIN)/4095 + I_MIN;
